simulink model "CryoDetXray"  (R2016b)
settings: Solver=ode45  StartTime=0.0  StopTime=10e-5  MaxStep=Tclk/4  RelTol=1e-3
values from neighbouring files (symbols this model uses):
  Fclk = Fadc    (= 307200000)    [setupCryoFPGAxray.m]
  Tclk = 1/Fclk    (= 3.25520833333e-09)    [setupCryoFPGAxray.m]
undefined symbols (not defined in the file or in its folder): AXI4, Lite, lpf, Naxi, xlipgetpartsetting
libraries: xbsIndex_r4 x1091, CryoDetLib x68, simulink x4, hdlsllib x1
(part 1 of 8)
settings Model: Creator=ssmith  LastModifiedBy=ssmith
settings DataIOCC: LimitDataPoints=on  SaveFormat=Array
settings OptimizationCC: BlockReduction=off  BooleanDataType=off  LifeSpan=inf
settings DebuggingCC: SaveWithParameterizedLinksMsg=none  UnderspecifiedInitializationDetection=Classic  MergeDetectMultiDrivingBlocksExec=none  SignalResolutionControl=TryResolveAllWithWarning  AllowSymbolicDim=off  SFUnexpectedBacktrackingDiag=warning  SFNoUnconditionalDefaultTransitionDiag=warning  SFExecutionAtInitializationDiag=none
settings HardwareCC: ProdBitPerPointer=32  ProdBitPerSizeT=32  ProdBitPerPtrDiffT=32  ProdLargestAtomicFloat=None  ProdIntDivRoundTo=Undefined  ProdEndianess=Unspecified  ProdWordSize=32  ProdHWDeviceType=32-bit Generic  TargetUnknown=on
settings ModelReferenceCC: PropagateSignalLabelsOutOfModel=off
settings GRTTargetCC: TargetLangStandard=C89/C90 (ANSI)  GeneratePreprocessorConditionals=Disable all
settings ConfigComp: CovMetricSettings=dw  CovHtmlReporting=on  CovSaveCumulativeToWorkspaceVar=on  CovSaveSingleToWorkspaceVar=on  CovExternalEMLEnable=off  CovSFcnEnable=off

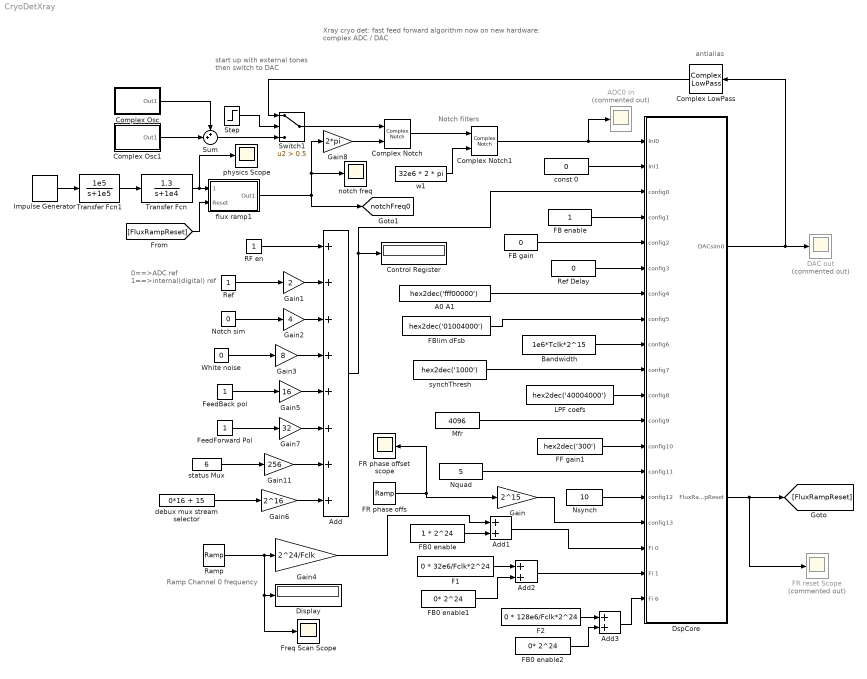
== system CryoDetXray ==
  note: antialias
  note: Ramp Channel 0 frequency
  note: Notch filters
  note: start up with external tones
      | then switch to DAC
  note: Xray cryo det: fast feed forward algorithm
      | now on new hardware:
      | complex ADC / DAC
  note: 0==>ADC ref
      | 1==>internal(digital) ref
  A0 A1 : Constant  Value=hex2dec('fff00000')  SampleTime=Tclk
  ADC0 in : Scope  Commented=on
  Add : Sum  Inputs=++++++++
  Add1 : Sum
  Add2 : Sum
  Add3 : Sum
  Bandwidth : Constant  Value=1e6*Tclk*2^15  SampleTime=Tclk
  Complex LowPass : CryoDetLib/Complex LowPass  num=lpf.num{1}  den=lpf.den{1}
  Complex Notch : CryoDetLib/Complex Notch  Q=16  depth=.95  Q1=10  depth1=1  Q2=10  depth2=1
  Complex Notch1 : CryoDetLib/Complex Notch  Q=8  depth=0.95  Q1=10  depth1=1  Q2=10  depth2=1
  Complex Osc : Subsystem  mask{Freq=64e6, Ampl=0.2}
  Complex Osc1 : Subsystem  mask{Freq=32e6, Ampl=0.2}
  Control Register : Display
      settings: Format=hex (Stored Integer)  Decimation=1000
  DAC out : Scope  Commented=on
  Display : Display
      settings: Decimation=64
  DspCore : Subsystem
  F1 : Constant  Value=0 * 32e6/Fclk*2^24  SampleTime=Tclk
  F2 : Constant  Value=0 * 128e6/Fclk*2^24  SampleTime=Tclk
  FB enable : Constant  SampleTime=Tclk
  FB gain : Constant  Value=0  SampleTime=Tclk
  FB0 enable : Constant  Value=1 * 2^24  SampleTime=Tclk
  FB0 enable1 : Constant  Value=0* 2^24  SampleTime=Tclk
  FB0 enable2 : Constant  Value=0* 2^24  SampleTime=Tclk
  FBlim dFsb : Constant  Value=hex2dec('01004000')  SampleTime=Tclk
  FF gain1 : Constant  Value=hex2dec('300')  SampleTime=Tclk
  FR phase offset scope : Scope
  FR phase offs : simulink/Sources/Ramp  slope=0/40e-5  start=26e-6  X0=.874
  FR reset Scope : Scope  Commented=on
  FeedBack pol : Constant  SampleTime=Tclk
  FeedForward Pol : Constant  SampleTime=Tclk
  Freq Scan Scope : Scope
  Gain : Gain  Gain=2^15
  Gain1 : Gain  Gain=2
  Gain11 : Gain  Gain=256
  Gain2 : Gain  Gain=4
  Gain3 : Gain  Gain=8
  Gain4 : Gain  Gain=2^24/Fclk
  Gain5 : Gain  Gain=16
  Gain6 : Gain  Gain=2^16
  Gain7 : Gain  Gain=32
  Gain8 : Gain  Gain=2*pi
  Impulse Generator : CryoDetLib/Impulse Generator  Impulse=1  width=2e-6  Period=1e-3  delay=15e-6
  LPF coefs : Constant  Value=hex2dec('40004000')  SampleTime=Tclk
  Mfr : Constant  Value=4096  SampleTime=Tclk
  Notch sim : Constant  Value=0  SampleTime=Tclk
  Nquad : Constant  Value=5  SampleTime=Tclk
  Nsynch : Constant  Value=10  SampleTime=Tclk
  RF en : Constant  SampleTime=Tclk
  Ramp : simulink/Sources/Ramp  slope=0 * 2e6/4e-6  start=1e-6  X0=64.0e6
  Ref : Constant  SampleTime=Tclk
  Ref Delay : Constant  Value=0  SampleTime=Tclk
  Step : Step  Time=2e-7  SampleTime=0
  Sum : Sum  Inputs=++|
  Switch1 : Switch  Criteria=u2 > Threshold  Threshold=0.5
  Transfer Fcn : TransferFcn  Numerator=[1.3]  Denominator=[1 1e4]
  Transfer Fcn1 : TransferFcn  Numerator=[1e5]  Denominator=[1 1e5]
  White noise : Constant  Value=0  SampleTime=Tclk
  const 0 : Constant  Value=0  SampleTime=Tclk
  debux mux stream selector : Constant  Value=0*16 + 15  SampleTime=Tclk
  flux ramp1 : Subsystem
  notch freq : Scope
  physics Scope : Scope
  status Mux : Constant  Value=6  SampleTime=Tclk
  synchThresh : Constant  Value=hex2dec('1000')  SampleTime=Tclk
  w1 : Constant  Value=32e6 * 2 * pi  SampleTime=Tclk
  tag scope: notchFreq0=global
  wires:
  Add/1 -> DspCore/3(config0), Control Register/1
  FB enable/1 -> DspCore/4(config1)
  DspCore/1(DACsim0) -> Complex LowPass/1, DAC out/1
  Sum/1 -> Switch1/3
  Step/1 -> Switch1/2
  RF en/1 -> Add/1
  Ref/1 -> Gain1/1
  Notch sim/1 -> Gain2/1
  White noise/1 -> Gain3/1
  FeedBack pol/1 -> Gain5/1
  debux mux stream selector/1 -> Gain6/1
  Gain1/1 -> Add/2
  Gain2/1 -> Add/3
  Gain3/1 -> Add/4
  status Mux/1 -> Gain11/1
  Complex Notch1/1 -> ADC0 in/1, DspCore/1(InI0)
  const 0/1 -> DspCore/2(InI1)
  Gain11/1 -> Add/7
  Gain6/1 -> Add/8
  Gain5/1 -> Add/5
  FB gain/1 -> DspCore/5(config2)
  Ref Delay/1 -> DspCore/6(config3)
  A0 A1/1 -> DspCore/7("config4 ")
  FBlim dFsb/1 -> DspCore/8(config5)
  Bandwidth/1 -> DspCore/9(config6)
  FeedForward Pol/1 -> Gain7/1
  FB0 enable/1 -> Add1/2
  Gain4/1 -> Add1/1
  Add1/1 -> DspCore/17(Fi 0)
  DspCore/2(FluxRampReset) -> [FluxRampReset], FR reset Scope/1
  Switch1/1 -> Complex Notch/1
  FB0 enable1/1 -> Add2/2
  F1/1 -> Add2/1
  Add2/1 -> DspCore/18(Fi 1)
  synchThresh/1 -> DspCore/10(config7)
  LPF coefs/1 -> DspCore/11(config8)
  FB0 enable2/1 -> Add3/2
  F2/1 -> Add3/1
  Add3/1 -> DspCore/19(Fi 6)
  Mfr/1 -> DspCore/12(config9)
  FF gain1/1 -> DspCore/13(config10)
  Nquad/1 -> DspCore/14(config11)
  Nsynch/1 -> DspCore/15(config12)
  Complex Osc1/1(Out1) -> Sum/2
  Complex Osc/1(Out1) -> Sum/1
  Gain8/1 -> Complex Notch/2
  w1/1 -> Complex Notch1/2
  [FluxRampReset] -> flux ramp1/2(Reset)
  Gain/1 -> DspCore/16(config13)
  Gain7/1 -> Add/6
  Ramp/1 -> Freq Scan Scope/1, Display/1, Gain4/1
  Impulse Generator/1 -> Transfer Fcn1/1
  Transfer Fcn/1 -> physics Scope/1, flux ramp1/1(physics)
  Complex LowPass/1 -> Switch1/1
  Complex Notch/1 -> Complex Notch1/1
  FR phase offs/1 -> Gain/1, FR phase offset scope/1
  flux ramp1/1(Out1) -> [notchFreq0], Gain8/1, notch freq/1
  Transfer Fcn1/1 -> Transfer Fcn/1

== system CryoDetXray/Complex Osc ==
  Cosine : Sin  Amplitude=Ampl  Frequency=2*pi*Freq  Phase=pi/2  SampleTime=0
  Real-Imag to Complex : RealImagToComplex
  Sine : Sin  Amplitude=Ampl  Frequency=2*pi*Freq  SampleTime=0
  Out1 : Outport
  wires:
  Real-Imag to Complex/1 -> Out1/1
  Cosine/1 -> Real-Imag to Complex/1
  Sine/1 -> Real-Imag to Complex/2

== system CryoDetXray/Complex Osc1 ==
  Cosine : Sin  Amplitude=Ampl  Frequency=2*pi*Freq  Phase=pi/2  SampleTime=0
  Real-Imag to Complex : RealImagToComplex
  Sine : Sin  Amplitude=Ampl  Frequency=2*pi*Freq  SampleTime=0
  Out1 : Outport
  wires:
  Real-Imag to Complex/1 -> Out1/1
  Cosine/1 -> Real-Imag to Complex/1
  Sine/1 -> Real-Imag to Complex/2

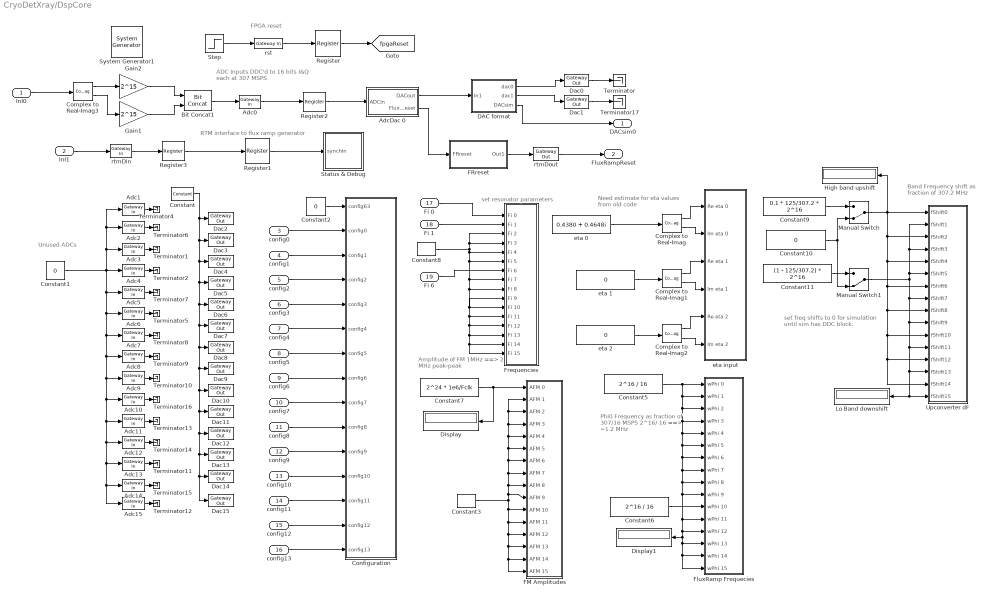
== system CryoDetXray/DspCore ==
  note: set freq shifts to 0 for simulation
      | until sim has DDC block.
  note: RTM interface to flux ramp generator
  note: Need estimate for eta values
      | from old code
  note: set resonator parameters
  note: Phi0 Frequency as fraction of 307/16 MSPS
      | 2^16/ 16 ==> ~1.2 MHz
  note: Amplitude of FM
      | 1MHz ==>
      | 2 MHz peak-peak
  note: Unused ADCs
  note: ADC Inputs DDC'd to
      | 16 bits I&Q each at 307 MSPS
  note: FPGA reset
  note: Band Frequency shift as fraction of 307.2 MHz
  InI0 : Inport
  InI1 : Inport  Port=2
  config0 : Inport  Port=3
  config1 : Inport  Port=4
  config2 : Inport  Port=5
  config3 : Inport  Port=6
  "config4 " : Inport  Port=7
  config5 : Inport  Port=8
  config6 : Inport  Port=9
  config7 : Inport  Port=10
  config8 : Inport  Port=11
  config9 : Inport  Port=12
  config10 : Inport  Port=13
  config11 : Inport  Port=14
  config12 : Inport  Port=15
  config13 : Inport  Port=16
  Fi 0 : Inport  Port=17
  Fi 1 : Inport  Port=18
  Fi 6 : Inport  Port=19
  " System Generator1" : xbsIndex_r4/ System Generator  Tag=genX  xilinxfamily=kintexu  part=xcku060  speed=-2-e  package=ffva1156  synthesis_tool=Vivado  clock_wrapper=Clock Enables  directory=./netlist  proj_type=Vivado  Synth_file=Vivado Synthesis Defaults  Impl_file=Vivado Implementation Defaults  testbench=off  simulink_period=Tclk  sysclk_period=Tclk*1e9  dcm_input_clock_period=10  incr_netlist=off  trim_vbits=Everywhere in SubSystem  dbl_ovrd=According to Block Masks  core_generation=According to Block Masks  run_coregen=off  deprecated_control=off  eval_field=0  block_type=sysgen
  Adc{0..15} (16 alike) : xbsIndex_r4/Gateway In  gui_display_data_type=Fixed-point  arith_type=Unsigned  n_bits=32  bin_pt=0  preci_type=Single  exp_width=8  frac_width=24  rows=1  columns=1  quantization=Truncate  overflow=Wrap  period=Ts  UseAsADC=off  ADCChannel='1'  interface=None  automatic_assignment=on  address_offset=hex2dec('00')  intf_name=''  intf_description=''  default_value=0  timing_constraint=None  locs_specified=off  LOCs={}  io_standard={}  inherit_from_input=off  hdl_port=on  dbl_ovrd=off  block_type=gatewayin
  AdcDac 0 : Subsystem
  Bit Concat1 : hdlsllib/HDL Operations/Bit Concat  numInputs=2
  Complex to Real-Imag{,1..3} (4 alike) : ComplexToRealImag
  Configuration : Subsystem
  Constant : xbsIndex_r4/Constant  const=0  gui_display_data_type=Fixed-point  arith_type=Unsigned  n_bits=32  bin_pt=0  preci_type=Single  exp_width=8  frac_width=24  explicit_period=off  period=1  equ=P=C  opselect=C  inp2=PCIN>>17  opr=+  inp1=P  carry=CIN  dbl_ovrd=off  block_type=constant
  Constant1 : Constant  Value=0
  Constant10 : Constant  Value=0
  Constant11 : Constant  Value=(1 - 125/307.2) * 2^16
  Constant2 : Constant  Value=0
  Constant3 : xbsIndex_r4/Constant  const=0  gui_display_data_type=Fixed-point  arith_type=Unsigned  n_bits=32  bin_pt=0  preci_type=Single  exp_width=8  frac_width=24  explicit_period=on  period=Tclk*Naxi  equ=P=C  opselect=C  inp2=PCIN>>17  opr=+  inp1=P  carry=CIN  dbl_ovrd=off  block_type=constant
  Constant5 : Constant  Value=2^16 / 16
  Constant6 : Constant  Value=2^16 / 16
  Constant7 : Constant  Value=2^24 * 1e6/Fclk
  Constant8 : xbsIndex_r4/Constant  const=0  gui_display_data_type=Fixed-point  arith_type=Unsigned  n_bits=32  bin_pt=0  preci_type=Single  exp_width=8  frac_width=24  explicit_period=on  period=Tclk*Naxi  equ=P=C  opselect=C  inp2=PCIN>>17  opr=+  inp1=P  carry=CIN  dbl_ovrd=off  block_type=constant
  Constant9 : Constant  Value="0.1  * 125/307.2 * 2^16"
  DAC format : Subsystem
  Dac{0,2..15} (15 alike) : xbsIndex_r4/Gateway Out  inherit_from_input=on  hdl_port=on  rows=1  columns=1  UseAsDAC=off  DACChannel='1'  interface=None  automatic_assignment=on  address_offset=hex2dec('00')  intf_name=''  intf_description=''  timing_constraint=None  locs_specified=off  LOCs={}  io_standard={}  block_type=gatewayout
  "Dac1 " : xbsIndex_r4/Gateway Out  inherit_from_input=on  hdl_port=on  rows=1  columns=1  UseAsDAC=off  DACChannel='1'  interface=None  automatic_assignment=on  address_offset=hex2dec('00')  intf_name=''  intf_description=''  timing_constraint=None  locs_specified=off  LOCs={}  io_standard={}  block_type=gatewayout
  Display : Display
  Display1 : Display
  FM Amplitudes : Subsystem
  FRreset : Subsystem
  FluxRamp Frequecies : Subsystem
  Frequencies : Subsystem
  Gain1 : Gain  Gain=2^15  OutDataTypeStr=int16  RndMeth=Nearest  SaturateOnIntegerOverflow=on
  Gain2 : Gain  Gain=2^15  OutDataTypeStr=int16  RndMeth=Nearest  SaturateOnIntegerOverflow=on
  High band upshift : Display
  Lo Band downshift : Display
  Manual Switch : ManualSwitch  CurrentSetting=0
  Manual Switch1 : ManualSwitch  CurrentSetting=0
  Register : xbsIndex_r4/Register  init=1  rst=off  en=off  dbl_ovrd=off  block_type=register
  Register1 : xbsIndex_r4/Register  init=1  rst=off  en=off  dbl_ovrd=off  block_type=register
  Register2 : xbsIndex_r4/Register  init=0  rst=off  en=off  dbl_ovrd=off  block_type=register
  Register3 : xbsIndex_r4/Register  init=0  rst=off  en=off  dbl_ovrd=off  block_type=register
  Status & Debug : Subsystem
  Step : Step  Time=1e-7  Before=1  After=0  SampleTime=0
  Terminator{,1..2,4..17} (17 alike) : Terminator
  Upconverter dF : Subsystem
  eta 0 : Constant  Value=0.4380 + 0.4648i
  eta 1 : Constant  Value=0
  "eta 2 " : Constant  Value=0
  eta input : Subsystem
  rst : xbsIndex_r4/Gateway In  gui_display_data_type=Boolean  arith_type=Boolean  n_bits=16  bin_pt=14  preci_type=Single  exp_width=8  frac_width=24  rows=1  columns=1  quantization="Round  (unbiased: +/- Inf)"  overflow=Saturate  period=Tclk  UseAsADC=off  ADCChannel='1'  interface=None  automatic_assignment=on  address_offset=hex2dec('00')  intf_name=''  intf_description=''  default_value=0  timing_constraint=None  locs_specified=off  LOCs={}  io_standard={}  inherit_from_input=off  hdl_port=on  dbl_ovrd=off  block_type=gatewayin
  rtmDin : xbsIndex_r4/Gateway In  gui_display_data_type=Fixed-point  arith_type=Unsigned  n_bits=16  bin_pt=0  preci_type=Single  exp_width=8  frac_width=24  rows=1  columns=1  quantization=Truncate  overflow=Wrap  period=Tclk  UseAsADC=off  ADCChannel='1'  interface=None  automatic_assignment=on  address_offset=hex2dec('00')  intf_name=''  intf_description=''  default_value=0  timing_constraint=None  locs_specified=off  LOCs={}  io_standard={}  inherit_from_input=off  hdl_port=on  dbl_ovrd=off  block_type=gatewayin
  rtmDout : xbsIndex_r4/Gateway Out  inherit_from_input=off  hdl_port=on  rows=1  columns=1  UseAsDAC=off  DACChannel='1'  interface=None  automatic_assignment=on  address_offset=hex2dec('00')  intf_name=''  intf_description=''  timing_constraint=None  locs_specified=off  LOCs={}  io_standard={}  block_type=gatewayout
  DACsim0 : Outport
  FluxRampReset : Outport  Port=2
  tag scope: fpgaReset=global
  wires:
  Step/1 -> rst/1
  rst/1 -> Register/1
  config0/1 -> Configuration/2(config0)
  config1/1 -> Configuration/3(config1)
  config2/1 -> Configuration/4(config2)
  config3/1 -> Configuration/5(config3)
  "config4 "/1 -> Configuration/6(config4)
  config5/1 -> Configuration/7(config5)
  config6/1 -> Configuration/8(config6)
  Fi 0/1 -> Frequencies/1("Fi 0 ")
  Register/1 -> [fpgaReset]
  Constant2/1 -> Configuration/1(config63)
  Fi 1/1 -> Frequencies/2(Fi 1)
  config7/1 -> Configuration/9(config7)
  config8/1 -> Configuration/10(config8)
  config9/1 -> Configuration/11(config9)
  config10/1 -> Configuration/12(config10)
  config11/1 -> Configuration/13(config11)
  config12/1 -> Configuration/14(config12)
  Constant8/1 -> Frequencies/3(Fi 2), Frequencies/4(Fi 3), Frequencies/16(Fi 15), Frequencies/15(Fi 14), Frequencies/14(Fi 13), Frequencies/13(Fi 12), Frequencies/12(Fi 11), Frequencies/11(Fi 10), Frequencies/10(Fi 9), Frequencies/9(Fi 8), Frequencies/8(Fi 7), Frequencies/6(Fi 5), Frequencies/5(Fi 4)
  Fi 6/1 -> Frequencies/7(Fi 6)
  AdcDac 0/2(FluxRampReset) -> FRreset/1(FRreset)
  Complex to Real-Imag/1 -> eta input/1(Re eta 0)
  Complex to Real-Imag/2 -> eta input/2(Im eta 0)
  Complex to Real-Imag1/1 -> eta input/3(Re eta 1)
  Complex to Real-Imag1/2 -> eta input/4(Im eta 1)
  eta 1/1 -> Complex to Real-Imag1/1
  Complex to Real-Imag2/1 -> eta input/5(Re eta 2)
  Complex to Real-Imag2/2 -> eta input/6(Im eta 2)
  "eta 2 "/1 -> Complex to Real-Imag2/1
  Constant6/1 -> FluxRamp Frequecies/11(wPhi 10)
  Constant7/1 -> Display/1, FM Amplitudes/1(AFM 0)
  Adc0/1 -> Register2/1
  FRreset/1(Out1) -> rtmDout/1
  Dac0/1 -> Terminator/1
  rtmDout/1 -> FluxRampReset/1
  Gain2/1 -> Bit Concat1/1
  Gain1/1 -> Bit Concat1/2
  Bit Concat1/1 -> Adc0/1
  config13/1 -> Configuration/15(config13)
  eta 0/1 -> Complex to Real-Imag/1
  Constant3/1 -> FM Amplitudes/11(AFM 10), FM Amplitudes/12(AFM 11), FM Amplitudes/13(AFM 12), FM Amplitudes/14(AFM 13), FM Amplitudes/15(AFM 14), FM Amplitudes/16(AFM 15), FM Amplitudes/10(AFM 9), FM Amplitudes/2(AFM 1), FM Amplitudes/3(AFM 2), FM Amplitudes/4(AFM 3), FM Amplitudes/5(AFM 4), FM Amplitudes/6(AFM 5), FM Amplitudes/7(AFM 6), FM Amplitudes/8(AFM 7), FM Amplitudes/9(AFM 8)
  Constant5/1 -> FluxRamp Frequecies/2(wPhi 1), FluxRamp Frequecies/3(wPhi 2), FluxRamp Frequecies/4(wPhi 3), FluxRamp Frequecies/5(wPhi 4), FluxRamp Frequecies/6(wPhi 5), FluxRamp Frequecies/7(wPhi 6), FluxRamp Frequecies/8(wPhi 7), FluxRamp Frequecies/13(wPhi 12), FluxRamp Frequecies/14(wPhi 13), FluxRamp Frequecies/15(wPhi 14), FluxRamp Frequecies/16(wPhi 15), Display1/1, FluxRamp Frequecies/12(wPhi 11), FluxRamp Frequecies/10(wPhi 9), FluxRamp Frequecies/9(wPhi 8), FluxRamp Frequecies/1(wPhi 0)
  Constant1/1 -> Adc5/1, Adc7/1, Adc8/1, Adc9/1, Adc10/1, Adc11/1, Adc12/1, Adc13/1, Adc14/1, Adc15/1, Adc6/1, Adc4/1, Adc3/1, Adc1/1, Adc2/1
  Complex to Real-Imag3/1 -> Gain2/1
  InI0/1 -> Complex to Real-Imag3/1
  Complex to Real-Imag3/2 -> Gain1/1
  InI1/1 -> rtmDin/1
  Adc6/1 -> Terminator5/1
  Adc7/1 -> Terminator8/1
  Adc8/1 -> Terminator9/1
  Adc9/1 -> Terminator10/1
  Adc11/1 -> Terminator13/1
  Adc12/1 -> Terminator14/1
  Adc13/1 -> Terminator11/1
  Adc14/1 -> Terminator15/1
  Adc15/1 -> Terminator12/1
  Adc10/1 -> Terminator16/1
  Adc1/1 -> Terminator4/1
  Adc2/1 -> Terminator6/1
  Adc3/1 -> Terminator1/1
  Adc4/1 -> Terminator2/1
  Adc5/1 -> Terminator7/1
  AdcDac 0/1(DACout) -> DAC format/1(In1)
  DAC format/3(DACsim) -> DACsim0/1
  DAC format/1(dac0) -> Dac0/1
  DAC format/2(dac1) -> "Dac1 "/1
  "Dac1 "/1 -> Terminator17/1
  Constant/1 -> Dac4/1, Dac5/1, Dac6/1, Dac7/1, Dac8/1, Dac9/1, Dac10/1, Dac11/1, Dac12/1, Dac13/1, Dac14/1, Dac15/1, Dac3/1, Dac2/1
  Manual Switch/1 -> Upconverter dF/1(fShift0), Upconverter dF/3(fShift2), Upconverter dF/5(fShift4), Upconverter dF/7(fShift6), Upconverter dF/11(fShift10), Upconverter dF/13(fShift12), Upconverter dF/15(fShift14), Upconverter dF/9(fShift8), High band upshift/1
  Constant9/1 -> Manual Switch/1
  Constant10/1 -> Manual Switch/2, Manual Switch1/2
  Constant11/1 -> Manual Switch1/1
  Manual Switch1/1 -> Upconverter dF/8(fShift7), Upconverter dF/10(fShift9), Upconverter dF/12(fShift11), Upconverter dF/14(fShift13), Lo Band downshift/1, Upconverter dF/16(fShift15), Upconverter dF/4(fShift3), Upconverter dF/2(fShift1), Upconverter dF/6(fShift5)
  rtmDin/1 -> Register3/1
  Register1/1 -> Status & Debug/1(synchIn)
  Register3/1 -> Register1/1
  Register2/1 -> AdcDac 0/1(ADCin)

== system CryoDetXray/flux ramp1 ==
  note: Simulate flux-ramp modulated center frequency of notch
      | with reset from flux ramp reset
  physics : Inport
  Reset : Inport  Port=2
  Add : Sum  Inputs=++|
  Add4 : Sum
  F1 : Constant  Value=307.2e6 / 16 / 16
  F3 : Constant  Value=64e6
  Integrator : Integrator  ExternalReset=rising
  Resonator w Flux Ramp Scope : Scope  Commented=on
  Resonator w Flux Ramp Scope1 : Scope  Commented=on
  Sine Wave : Sin  TimeSource=Use external signal  Amplitude=1e6  Frequency=2*pi  SampleTime=0
  Out1 : Outport
  wires:
  Add4/1 -> Resonator w Flux Ramp Scope/1, Out1/1
  F3/1 -> Add4/2
  F1/1 -> Integrator/1
  Reset/1 -> Integrator/2
  Sine Wave/1 -> Add4/1
  Integrator/1 -> Add/2
  Add/1 -> Resonator w Flux Ramp Scope1/1, Sine Wave/1
  physics/1 -> Add/1

== system CryoDetXray/DspCore/AdcDac 0 ==
  note: commented out 7 Oct 2017 as LR says number of logic level too much for router
  note: Does NOT work yet
      | 26 Sep 2017
  note: loop filter for loop which feeds back on
      | phase of flux ramp
  note: Estimate FluxRamp Phase
  note: Estimate frequency error at high bandwidth
  note: freqBusHBW goes to DDS to generate output tones
      | FR reset goes to flux ramp function generator
  note: loop filter output will be mux'd channel, fluix ramp phase shift
  note: High bandwidth/ no sideband scheme
  note: Low Bandwidth / +- sideband scheme
      | (but sideband generator has been removed)
  note: 9 June SRS pulled LPF out of eta subsytem
      | so that amplitudes subsystem can use low-pass filtered I&Q data
      | Also added Signal central line to LPF processing as Amplitudes block uses it, though eta does not
  ADCin : Inport
  16LineUDC 0 : Subsystem
  16LineUDC 1 : Subsystem
  16ch LBW LPF : Subsystem
  Amplitudes : Subsystem
  Bus Creator : BusCreator  Inputs=2
  Bus Selector : BusSelector  Commented=on  OutputSignals=channel,Sig&Ref.SignalQ&I.sigQ,Sig&Ref.SignalQ&I.sigI,Sig&Ref.ReferenceQ&I.refQ,Sig&Ref.ReferenceQ&I.refI
  "Flux Ramp DDC " : Subsystem
  FluxRamp : Subsystem
  Gateway Out{1..3,5..6} (5 alike) : xbsIndex_r4/Gateway Out  Commented=on  inherit_from_input=off  hdl_port=off  rows=1  columns=1  UseAsDAC=off  DACChannel='1'  interface=None  automatic_assignment=on  address_offset=hex2dec('00')  intf_name=''  intf_description=''  timing_constraint=None  locs_specified=off  LOCs={}  io_standard={}  block_type=gatewayout
  HBW Sig/Ref LPF : Subsystem  Commented=on
  Mux : Mux  Commented=on  Inputs=2
  Mux1 : Mux  Commented=on  Inputs=2
  RF switch : Subsystem
  Ref Delay : Subsystem
  S21 : Subsystem  Commented=on
  SigXrefIQ : Scope  Commented=on  NumInputPorts=3
  Terminator : Terminator
  Terminator2 : Terminator  Commented=on
  Terminator3 : Terminator  Commented=on
  dF1 : Subsystem
  dphi : Subsystem
  loopFilter1 : Subsystem
  shiftFreq : Subsystem
  DACout : Outport
  FluxRampReset : Outport  Port=2
  tag scope: freqBusHBW=global
  wires:
  16LineUDC 1/1(Out1) -> Terminator/1
  16LineUDC 0/1(toDAC) -> RF switch/1(In1)
  ADCin/1 -> Bus Creator/1  "ADCin"
  Ref Delay/1(Out1) -> Bus Creator/2
  Bus Creator/1 -> 16LineUDC 1/1(In1), 16LineUDC 0/1(In1)
  16LineUDC 0/2(demodulated) -> 16ch LBW LPF/1(In1)
  RF switch/1(Out1) -> Ref Delay/1(In1), shiftFreq/1(In1)
  16ch LBW LPF/1(Out1) -> Amplitudes/1(In2)
  16LineUDC 0/3(hiBW) -> Bus Selector/1, HBW Sig/Ref LPF/1(In1), dF1/1(In1)
  HBW Sig/Ref LPF/1(Out1) -> S21/1(In2)
  loopFilter1/1(Out1) -> FluxRamp/1(phiFR)
  "Flux Ramp DDC "/1(Out1) -> loopFilter1/1(In1)
  FluxRamp/2(freqBusHBW) -> [freqBusHBW]
  FluxRamp/4(FiBus) -> dphi/1(In1)
  FluxRamp/3(FR reset) -> FluxRampReset/1
  S21/1(S21Bus) -> Terminator2/1
  S21/2(S21BusLPF) -> Terminator3/1
  dF1/1(Out1) -> "Flux Ramp DDC "/1(FreqErrIn)
  FluxRamp/1(FluxRampLO) -> "Flux Ramp DDC "/2(FluxRampLO)
  shiftFreq/1(Out1) -> DACout/1
  Gateway Out5/1 -> Mux/1
  Gateway Out6/1 -> Mux/2
  Gateway Out2/1 -> Mux1/2
  Gateway Out1/1 -> Mux1/1
  Gateway Out3/1 -> SigXrefIQ/1
  Mux/1 -> SigXrefIQ/2
  Mux1/1 -> SigXrefIQ/3
  Bus Selector/1 -> Gateway Out3/1  "<channel>"
  Bus Selector/2 -> Gateway Out5/1  "<sigQ>"
  Bus Selector/3 -> Gateway Out6/1  "<sigI>"
  Bus Selector/4 -> Gateway Out1/1  "<refQ>"
  Bus Selector/5 -> Gateway Out2/1  "<refI>"

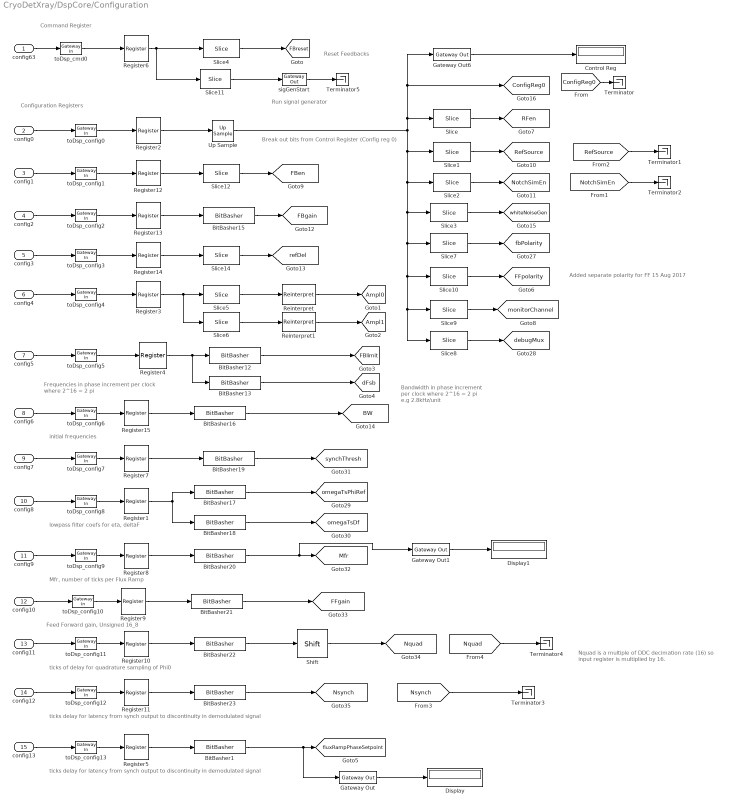
== system CryoDetXray/DspCore/Configuration ==
  note: Run signal generator
  note: Reset Feedbacks
  note: Nquad is a multiple of DDC decimation rate (16)
      | so input register is multiplied by 16.
  note: Added separate polarity for FF 15 Aug 2017
  note: Frequencies in phase increment per clock
      | where 2^16 = 2 pi
  note: initial frequencies
  note: Configuration Registers
  note: Command Register
  note: Break out bits from Control Register (Config reg 0)
  note: Bandwidth in phase increment per clock
      | where 2^16 = 2 pi e.g 2.8kHz/unit
  note: lowpass filter coefs for eta, deltaF
  note: Mfr, number of ticks per Flux Ramp
  note: Feed Forward gain, Unsigned 16_8
  note: ticks of delay for quadrature sampling of Phi0
  note: ticks delay for latency from synch output to discontinuity in demodulated signal
  note: ticks delay for latency from synch output to discontinuity in demodulated signal
  config63 : Inport
  config0 : Inport  Port=2
  config1 : Inport  Port=3
  config2 : Inport  Port=4
  config3 : Inport  Port=5
  config4 : Inport  Port=6
  config5 : Inport  Port=7
  config6 : Inport  Port=8
  config7 : Inport  Port=9
  config8 : Inport  Port=10
  config9 : Inport  Port=11
  config10 : Inport  Port=12
  config11 : Inport  Port=13
  config12 : Inport  Port=14
  config13 : Inport  Port=15
  BitBasher1 : xbsIndex_r4/BitBasher  bitexpr=a={b[15:0]}  display_expr=on  sr_1=a  arith_type1="Signed  (2's comp)"  bin_pt1=15  sr_2=2  arith_type2=Unsigned  bin_pt2=0  sr_3=3  arith_type3=Unsigned  bin_pt3=0  sr_4=4  arith_type4=Unsigned  bin_pt4=0  dbl_ovrd=off  block_type=bitbasher
  BitBasher12 : xbsIndex_r4/BitBasher  bitexpr=a={b[31:16]}  display_expr=on  sr_1=a  arith_type1=Unsigned  bin_pt1=16  sr_2=2  arith_type2=Unsigned  bin_pt2=0  sr_3=3  arith_type3=Unsigned  bin_pt3=0  sr_4=4  arith_type4=Unsigned  bin_pt4=0  dbl_ovrd=off  block_type=bitbasher
  BitBasher13 : xbsIndex_r4/BitBasher  bitexpr=a={b[15:0]}  display_expr=on  sr_1=a  arith_type1=Unsigned  bin_pt1=16  sr_2=2  arith_type2=Unsigned  bin_pt2=0  sr_3=3  arith_type3=Unsigned  bin_pt3=0  sr_4=4  arith_type4=Unsigned  bin_pt4=0  dbl_ovrd=off  block_type=bitbasher
  BitBasher15 : xbsIndex_r4/BitBasher  bitexpr=a={b[15:0]}  display_expr=on  sr_1=a  arith_type1=Unsigned  bin_pt1=12  sr_2=2  arith_type2=Unsigned  bin_pt2=0  sr_3=3  arith_type3=Unsigned  bin_pt3=0  sr_4=4  arith_type4=Unsigned  bin_pt4=0  dbl_ovrd=off  block_type=bitbasher
  BitBasher16 : xbsIndex_r4/BitBasher  bitexpr=a={b[15:0]}  display_expr=on  sr_1=a  arith_type1="Signed  (2's comp)"  bin_pt1=15  sr_2=2  arith_type2=Unsigned  bin_pt2=0  sr_3=3  arith_type3=Unsigned  bin_pt3=0  sr_4=4  arith_type4=Unsigned  bin_pt4=0  dbl_ovrd=off  block_type=bitbasher
  BitBasher17 : xbsIndex_r4/BitBasher  bitexpr=a={b[15:0]}  display_expr=on  sr_1=a  arith_type1=Unsigned  bin_pt1=16  sr_2=2  arith_type2=Unsigned  bin_pt2=0  sr_3=3  arith_type3=Unsigned  bin_pt3=0  sr_4=4  arith_type4=Unsigned  bin_pt4=0  dbl_ovrd=off  block_type=bitbasher
  BitBasher18 : xbsIndex_r4/BitBasher  bitexpr=a={b[31:16]}  display_expr=on  sr_1=a  arith_type1=Unsigned  bin_pt1=16  sr_2=2  arith_type2=Unsigned  bin_pt2=0  sr_3=3  arith_type3=Unsigned  bin_pt3=0  sr_4=4  arith_type4=Unsigned  bin_pt4=0  dbl_ovrd=off  block_type=bitbasher
  BitBasher19 : xbsIndex_r4/BitBasher  bitexpr=a={b[15:0]}  display_expr=on  sr_1=a  arith_type1="Signed  (2's comp)"  bin_pt1=15  sr_2=2  arith_type2=Unsigned  bin_pt2=0  sr_3=3  arith_type3=Unsigned  bin_pt3=0  sr_4=4  arith_type4=Unsigned  bin_pt4=0  dbl_ovrd=off  block_type=bitbasher
  BitBasher20 : xbsIndex_r4/BitBasher  bitexpr=a={b[15:0]}  display_expr=on  sr_1=a  arith_type1=Unsigned  bin_pt1=0  sr_2=2  arith_type2=Unsigned  bin_pt2=0  sr_3=3  arith_type3=Unsigned  bin_pt3=0  sr_4=4  arith_type4=Unsigned  bin_pt4=0  dbl_ovrd=off  block_type=bitbasher
  BitBasher21 : xbsIndex_r4/BitBasher  bitexpr=a={b[15:0]}  display_expr=on  sr_1=a  arith_type1=Unsigned  bin_pt1=4  sr_2=2  arith_type2=Unsigned  bin_pt2=0  sr_3=3  arith_type3=Unsigned  bin_pt3=0  sr_4=4  arith_type4=Unsigned  bin_pt4=0  dbl_ovrd=off  block_type=bitbasher
  BitBasher22 : xbsIndex_r4/BitBasher  bitexpr=a={b[3:0]}  display_expr=on  sr_1=a  arith_type1=Unsigned  bin_pt1=0  sr_2=2  arith_type2=Unsigned  bin_pt2=0  sr_3=3  arith_type3=Unsigned  bin_pt3=0  sr_4=4  arith_type4=Unsigned  bin_pt4=0  dbl_ovrd=off  block_type=bitbasher
  BitBasher23 : xbsIndex_r4/BitBasher  bitexpr=a={b[7:0]}  display_expr=on  sr_1=a  arith_type1=Unsigned  bin_pt1=0  sr_2=2  arith_type2=Unsigned  bin_pt2=0  sr_3=3  arith_type3=Unsigned  bin_pt3=0  sr_4=4  arith_type4=Unsigned  bin_pt4=0  dbl_ovrd=off  block_type=bitbasher
  Control Reg : Display
  Display : Display
  Display1 : Display
  Gateway Out : xbsIndex_r4/Gateway Out  inherit_from_input=off  hdl_port=off  rows=1  columns=1  UseAsDAC=off  DACChannel='1'  interface=None  automatic_assignment=on  address_offset=hex2dec('00')  intf_name=''  intf_description=''  timing_constraint=None  locs_specified=off  LOCs={}  io_standard={}  block_type=gatewayout
  Gateway Out1 : xbsIndex_r4/Gateway Out  inherit_from_input=off  hdl_port=off  rows=1  columns=1  UseAsDAC=off  DACChannel='1'  interface=None  automatic_assignment=on  address_offset=hex2dec('00')  intf_name=''  intf_description=''  timing_constraint=None  locs_specified=off  LOCs={}  io_standard={}  block_type=gatewayout
  Gateway Out6 : xbsIndex_r4/Gateway Out  inherit_from_input=off  hdl_port=off  rows=1  columns=1  UseAsDAC=off  DACChannel='1'  interface=None  automatic_assignment=on  address_offset=hex2dec('00')  intf_name=''  intf_description=''  timing_constraint=None  locs_specified=off  LOCs={}  io_standard={}  block_type=gatewayout
  Register{1..15} (15 alike) : xbsIndex_r4/Register  init=0  rst=off  en=off  dbl_ovrd=off  block_type=register
  Reinterpret : xbsIndex_r4/Reinterpret  force_arith_type=on  arith_type=Unsigned  force_bin_pt=on  bin_pt=16  block_type=reinterpret
  Reinterpret1 : xbsIndex_r4/Reinterpret  force_arith_type=on  arith_type=Unsigned  force_bin_pt=on  bin_pt=16  block_type=reinterpret
  Shift : xbsIndex_r4/Shift  shift_dir=Left  shift_bits=4  en=off  latency=1  precision=User Defined  arith_type=Unsigned  n_bits=8  bin_pt=0  quantization=Truncate  overflow=Wrap  dbl_ovrd=off  block_type=shift
  Slice : xbsIndex_r4/Slice  nbits=1  boolean_output=off  mode=Upper Bit Location + Width  bit1=0  base1=LSB of Input  bit0=0  base0=LSB of Input  dbl_ovrd=off  block_type=slice
  Slice1 : xbsIndex_r4/Slice  nbits=1  boolean_output=on  mode=Upper Bit Location + Width  bit1=1  base1=LSB of Input  bit0=0  base0=LSB of Input  dbl_ovrd=off  block_type=slice
  Slice10 : xbsIndex_r4/Slice  nbits=1  boolean_output=on  mode=Upper Bit Location + Width  bit1=5  base1=LSB of Input  bit0=0  base0=LSB of Input  dbl_ovrd=off  block_type=slice
  Slice11 : xbsIndex_r4/Slice  nbits=1  boolean_output=on  mode=Upper Bit Location + Width  bit1=4  base1=LSB of Input  bit0=0  base0=LSB of Input  dbl_ovrd=off  block_type=slice
  Slice12 : xbsIndex_r4/Slice  nbits=1  boolean_output=on  mode=Upper Bit Location + Width  bit1=0  base1=LSB of Input  bit0=0  base0=LSB of Input  dbl_ovrd=off  block_type=slice
  Slice14 : xbsIndex_r4/Slice  nbits=8  boolean_output=off  mode=Lower Bit Location + Width  bit1=0  base1=LSB of Input  bit0=0  base0=LSB of Input  dbl_ovrd=off  block_type=slice
  Slice2 : xbsIndex_r4/Slice  nbits=1  boolean_output=on  mode=Upper Bit Location + Width  bit1=2  base1=LSB of Input  bit0=0  base0=LSB of Input  dbl_ovrd=off  block_type=slice
  Slice3 : xbsIndex_r4/Slice  nbits=1  boolean_output=on  mode=Upper Bit Location + Width  bit1=3  base1=LSB of Input  bit0=0  base0=LSB of Input  dbl_ovrd=off  block_type=slice
  Slice4 : xbsIndex_r4/Slice  nbits=1  boolean_output=on  mode=Upper Bit Location + Width  bit1=0  base1=LSB of Input  bit0=0  base0=LSB of Input  dbl_ovrd=off  block_type=slice
  Slice5 : xbsIndex_r4/Slice  nbits=16  boolean_output=off  mode=Upper Bit Location + Width  bit1=31  base1=LSB of Input  bit0=0  base0=LSB of Input  dbl_ovrd=off  block_type=slice
  Slice6 : xbsIndex_r4/Slice  nbits=16  boolean_output=off  mode=Upper Bit Location + Width  bit1=15  base1=LSB of Input  bit0=0  base0=LSB of Input  dbl_ovrd=off  block_type=slice
  Slice7 : xbsIndex_r4/Slice  nbits=1  boolean_output=on  mode=Upper Bit Location + Width  bit1=4  base1=LSB of Input  bit0=0  base0=LSB of Input  dbl_ovrd=off  block_type=slice
  Slice8 : xbsIndex_r4/Slice  nbits=8  boolean_output=off  mode=Lower Bit Location + Width  bit1=6  base1=LSB of Input  bit0=16  base0=LSB of Input  dbl_ovrd=off  block_type=slice
  Slice9 : xbsIndex_r4/Slice  nbits=8  boolean_output=off  mode=Lower Bit Location + Width  bit1=6  base1=LSB of Input  bit0=8  base0=LSB of Input  dbl_ovrd=off  block_type=slice
  Terminator{,1..5} (6 alike) : Terminator
  Up Sample : xbsIndex_r4/Up Sample  sample_ratio=Naxi  copy_samples=on  en=off  latency=1  dbl_ovrd=off  block_type=usamp
  sigGenStart : xbsIndex_r4/Gateway Out  inherit_from_input=on  hdl_port=on  rows=1  columns=1  UseAsDAC=off  DACChannel='1'  interface=None  automatic_assignment=off  address_offset=hex2dec('004')  intf_name=''  intf_description=''  timing_constraint=None  locs_specified=off  LOCs={}  io_standard={}  block_type=gatewayout
  toDsp_cmd0 : xbsIndex_r4/Gateway In  gui_display_data_type=Fixed-point  arith_type=Unsigned  n_bits=32  bin_pt=0  preci_type=Single  exp_width=8  frac_width=24  rows=1  columns=1  quantization=Truncate  overflow=Wrap  period=Tclk*Naxi  UseAsADC=off  ADCChannel='1'  interface=AXI4-Lite  automatic_assignment=off  address_offset=hex2dec('8fc')  intf_name=''  intf_description=''  default_value=0  timing_constraint=None  locs_specified=off  LOCs={}  io_standard={}  inherit_from_input=off  hdl_port=on  dbl_ovrd=off  block_type=gatewayin
  toDsp_config0 : xbsIndex_r4/Gateway In  gui_display_data_type=Fixed-point  arith_type=Unsigned  n_bits=32  bin_pt=0  preci_type=Single  exp_width=8  frac_width=24  rows=1  columns=1  quantization=Truncate  overflow=Wrap  period=Tclk*Naxi  UseAsADC=off  ADCChannel='1'  interface=AXI4-Lite  automatic_assignment=off  address_offset=hex2dec('800')  intf_name=''  intf_description=''  default_value=0  timing_constraint=None  locs_specified=off  LOCs={}  io_standard={}  inherit_from_input=off  hdl_port=on  dbl_ovrd=off  block_type=gatewayin
  toDsp_config1 : xbsIndex_r4/Gateway In  gui_display_data_type=Fixed-point  arith_type=Unsigned  n_bits=32  bin_pt=0  preci_type=Single  exp_width=8  frac_width=24  rows=1  columns=1  quantization=Truncate  overflow=Wrap  period=Tclk*Naxi  UseAsADC=off  ADCChannel='1'  interface=AXI4-Lite  automatic_assignment=off  address_offset=hex2dec('804')  intf_name=''  intf_description=''  default_value=0  timing_constraint=None  locs_specified=off  LOCs={}  io_standard={}  inherit_from_input=off  hdl_port=on  dbl_ovrd=off  block_type=gatewayin
  toDsp_config10 : xbsIndex_r4/Gateway In  gui_display_data_type=Fixed-point  arith_type=Unsigned  n_bits=32  bin_pt=0  preci_type=Single  exp_width=8  frac_width=24  rows=1  columns=1  quantization=Truncate  overflow=Wrap  period=Tclk*Naxi  UseAsADC=off  ADCChannel='1'  interface=AXI4-Lite  automatic_assignment=off  address_offset=hex2dec('828')  intf_name=''  intf_description=''  default_value=0  timing_constraint=None  locs_specified=off  LOCs={}  io_standard={}  inherit_from_input=off  hdl_port=on  dbl_ovrd=off  block_type=gatewayin
  toDsp_config11 : xbsIndex_r4/Gateway In  gui_display_data_type=Fixed-point  arith_type=Unsigned  n_bits=32  bin_pt=0  preci_type=Single  exp_width=8  frac_width=24  rows=1  columns=1  quantization=Truncate  overflow=Wrap  period=Tclk*Naxi  UseAsADC=off  ADCChannel='1'  interface=AXI4-Lite  automatic_assignment=off  address_offset=hex2dec('82c')  intf_name=''  intf_description=''  default_value=0  timing_constraint=None  locs_specified=off  LOCs={}  io_standard={}  inherit_from_input=off  hdl_port=on  dbl_ovrd=off  block_type=gatewayin
  toDsp_config12 : xbsIndex_r4/Gateway In  gui_display_data_type=Fixed-point  arith_type=Unsigned  n_bits=32  bin_pt=0  preci_type=Single  exp_width=8  frac_width=24  rows=1  columns=1  quantization=Truncate  overflow=Wrap  period=Tclk*Naxi  UseAsADC=off  ADCChannel='1'  interface=AXI4-Lite  automatic_assignment=off  address_offset=hex2dec('830')  intf_name=''  intf_description=''  default_value=0  timing_constraint=None  locs_specified=off  LOCs={}  io_standard={}  inherit_from_input=off  hdl_port=on  dbl_ovrd=off  block_type=gatewayin
  toDsp_config13 : xbsIndex_r4/Gateway In  gui_display_data_type=Fixed-point  arith_type=Unsigned  n_bits=32  bin_pt=0  preci_type=Single  exp_width=8  frac_width=24  rows=1  columns=1  quantization=Truncate  overflow=Wrap  period=Tclk*Naxi  UseAsADC=off  ADCChannel='1'  interface=AXI4-Lite  automatic_assignment=off  address_offset=hex2dec('834')  intf_name=''  intf_description=''  default_value=0  timing_constraint=None  locs_specified=off  LOCs={}  io_standard={}  inherit_from_input=off  hdl_port=on  dbl_ovrd=off  block_type=gatewayin
  toDsp_config2 : xbsIndex_r4/Gateway In  gui_display_data_type=Fixed-point  arith_type=Unsigned  n_bits=32  bin_pt=12  preci_type=Single  exp_width=8  frac_width=24  rows=1  columns=1  quantization=Truncate  overflow=Wrap  period=Tclk*Naxi  UseAsADC=off  ADCChannel='1'  interface=AXI4-Lite  automatic_assignment=off  address_offset=hex2dec('808')  intf_name=''  intf_description=''  default_value=0  timing_constraint=None  locs_specified=off  LOCs={}  io_standard={}  inherit_from_input=off  hdl_port=on  dbl_ovrd=off  block_type=gatewayin
  toDsp_config3 : xbsIndex_r4/Gateway In  gui_display_data_type=Fixed-point  arith_type=Unsigned  n_bits=32  bin_pt=0  preci_type=Single  exp_width=8  frac_width=24  rows=1  columns=1  quantization=Truncate  overflow=Wrap  period=Tclk*Naxi  UseAsADC=off  ADCChannel='1'  interface=AXI4-Lite  automatic_assignment=off  address_offset=hex2dec('80c')  intf_name=''  intf_description=''  default_value=0  timing_constraint=None  locs_specified=off  LOCs={}  io_standard={}  inherit_from_input=off  hdl_port=on  dbl_ovrd=off  block_type=gatewayin
  toDsp_config4 : xbsIndex_r4/Gateway In  gui_display_data_type=Fixed-point  arith_type=Unsigned  n_bits=32  bin_pt=0  preci_type=Single  exp_width=8  frac_width=24  rows=1  columns=1  quantization=Truncate  overflow=Wrap  period=Tclk*Naxi  UseAsADC=off  ADCChannel='1'  interface=AXI4-Lite  automatic_assignment=off  address_offset=hex2dec('810')  intf_name=''  intf_description=''  default_value=0  timing_constraint=None  locs_specified=off  LOCs={}  io_standard={}  inherit_from_input=off  hdl_port=on  dbl_ovrd=off  block_type=gatewayin
  toDsp_config5 : xbsIndex_r4/Gateway In  gui_display_data_type=Fixed-point  arith_type=Unsigned  n_bits=32  bin_pt=0  preci_type=Single  exp_width=8  frac_width=24  rows=1  columns=1  quantization=Truncate  overflow=Wrap  period=Tclk*Naxi  UseAsADC=off  ADCChannel='1'  interface=AXI4-Lite  automatic_assignment=off  address_offset=hex2dec('814')  intf_name=''  intf_description=''  default_value=0  timing_constraint=None  locs_specified=off  LOCs={}  io_standard={}  inherit_from_input=off  hdl_port=on  dbl_ovrd=off  block_type=gatewayin
  toDsp_config6 : xbsIndex_r4/Gateway In  gui_display_data_type=Fixed-point  arith_type=Unsigned  n_bits=32  bin_pt=0  preci_type=Single  exp_width=8  frac_width=24  rows=1  columns=1  quantization=Truncate  overflow=Wrap  period=Tclk*Naxi  UseAsADC=off  ADCChannel='1'  interface=AXI4-Lite  automatic_assignment=off  address_offset=hex2dec('818')  intf_name=''  intf_description=''  default_value=0  timing_constraint=None  locs_specified=off  LOCs={}  io_standard={}  inherit_from_input=off  hdl_port=on  dbl_ovrd=off  block_type=gatewayin
  toDsp_config7 : xbsIndex_r4/Gateway In  gui_display_data_type=Fixed-point  arith_type="Signed  (2's comp)"  n_bits=32  bin_pt=0  preci_type=Single  exp_width=8  frac_width=24  rows=1  columns=1  quantization=Truncate  overflow=Wrap  period=Tclk*Naxi  UseAsADC=off  ADCChannel='1'  interface=AXI4-Lite  automatic_assignment=off  address_offset=hex2dec('81c')  intf_name=''  intf_description=''  default_value=0  timing_constraint=None  locs_specified=off  LOCs={}  io_standard={}  inherit_from_input=off  hdl_port=on  dbl_ovrd=off  block_type=gatewayin
  toDsp_config8 : xbsIndex_r4/Gateway In  gui_display_data_type=Fixed-point  arith_type=Unsigned  n_bits=32  bin_pt=0  preci_type=Single  exp_width=8  frac_width=24  rows=1  columns=1  quantization=Truncate  overflow=Wrap  period=Tclk*Naxi  UseAsADC=off  ADCChannel='1'  interface=AXI4-Lite  automatic_assignment=off  address_offset=hex2dec('820')  intf_name=''  intf_description=''  default_value=0  timing_constraint=None  locs_specified=off  LOCs={}  io_standard={}  inherit_from_input=off  hdl_port=on  dbl_ovrd=off  block_type=gatewayin
  toDsp_config9 : xbsIndex_r4/Gateway In  gui_display_data_type=Fixed-point  arith_type=Unsigned  n_bits=32  bin_pt=0  preci_type=Single  exp_width=8  frac_width=24  rows=1  columns=1  quantization=Truncate  overflow=Wrap  period=Tclk*Naxi  UseAsADC=off  ADCChannel='1'  interface=AXI4-Lite  automatic_assignment=off  address_offset=hex2dec('824')  intf_name=''  intf_description=''  default_value=0  timing_constraint=None  locs_specified=off  LOCs={}  io_standard={}  inherit_from_input=off  hdl_port=on  dbl_ovrd=off  block_type=gatewayin
  tag scope: Ampl0=global, Ampl1=global, BW=global, ConfigReg0=global, FBen=global, FBgain=global, FBlimit=global, FBreset=global, FFgain=global, FFpolarity=global, Mfr=global, NotchSimEn=global, Nquad=global, Nsynch=global, RFen=global, RefSource=global, dFsb=global, debugMux=global, fbPolarity=global, fluxRampPhaseSetpoint=global, monitorChannel=global, omegaTsDf=global, omegaTsPhiRef=global, refDel=global, synchThresh=global, whiteNoiseGen=global
  wires:
  config0/1 -> toDsp_config0/1
  toDsp_config0/1 -> Register2/1
  config4/1 -> toDsp_config4/1
  toDsp_config4/1 -> Register3/1
  config5/1 -> toDsp_config5/1
  toDsp_config5/1 -> Register4/1
  config63/1 -> toDsp_cmd0/1
  toDsp_cmd0/1 -> Register6/1
  Register3/1 -> Slice6/1, Slice5/1
  Register6/1 -> Slice11/1, Slice4/1
  Slice5/1 -> Reinterpret/1
  Slice6/1 -> Reinterpret1/1
  Register4/1 -> BitBasher13/1, BitBasher12/1
  Slice1/1 -> [RefSource]
  Slice/1 -> [RFen]
  Slice2/1 -> [NotchSimEn]
  Slice3/1 -> [whiteNoiseGen]
  Reinterpret/1 -> [Ampl0]
  Reinterpret1/1 -> [Ampl1]
  Gateway Out6/1 -> Control Reg/1
  Slice4/1 -> [FBreset]
  BitBasher13/1 -> [dFsb]
  BitBasher12/1 -> [FBlimit]
  [NotchSimEn] -> Terminator2/1
  Slice9/1 -> [monitorChannel]
  config1/1 -> toDsp_config1/1
  toDsp_config1/1 -> Register12/1
  config2/1 -> toDsp_config2/1
  toDsp_config2/1 -> Register13/1
  config3/1 -> toDsp_config3/1
  toDsp_config3/1 -> Register14/1
  Slice12/1 -> [FBen]
  Register12/1 -> Slice12/1
  BitBasher15/1 -> [FBgain]
  Register13/1 -> BitBasher15/1
  Slice14/1 -> [refDel]
  Register14/1 -> Slice14/1
  config6/1 -> toDsp_config6/1
  toDsp_config6/1 -> Register15/1
  Register15/1 -> BitBasher16/1
  Slice7/1 -> [fbPolarity]
  [RefSource] -> Terminator1/1
  Slice8/1 -> [debugMux]
  BitBasher16/1 -> [BW]
  toDsp_config8/1 -> Register1/1
  Register1/1 -> BitBasher17/1, BitBasher18/1
  BitBasher17/1 -> [omegaTsPhiRef]
  BitBasher18/1 -> [omegaTsDf]
  config8/1 -> toDsp_config8/1
  toDsp_config7/1 -> Register7/1
  Register7/1 -> BitBasher19/1
  config7/1 -> toDsp_config7/1
  BitBasher19/1 -> [synchThresh]
  [ConfigReg0] -> Terminator/1
  toDsp_config9/1 -> Register8/1
  Register8/1 -> BitBasher20/1
  BitBasher20/1 -> Gateway Out1/1, [Mfr]
  config9/1 -> toDsp_config9/1
  toDsp_config10/1 -> Register9/1
  Register9/1 -> BitBasher21/1
  BitBasher21/1 -> [FFgain]
  config10/1 -> toDsp_config10/1
  toDsp_config11/1 -> Register10/1
  Register10/1 -> BitBasher22/1
  config11/1 -> toDsp_config11/1
  toDsp_config12/1 -> Register11/1
  Register11/1 -> BitBasher23/1
  BitBasher23/1 -> [Nsynch]
  config12/1 -> toDsp_config12/1
  [Nsynch] -> Terminator3/1
  BitBasher22/1 -> Shift/1
  Shift/1 -> [Nquad]
  [Nquad] -> Terminator4/1
  toDsp_config13/1 -> Register5/1
  Register5/1 -> BitBasher1/1
  BitBasher1/1 -> Gateway Out/1, [fluxRampPhaseSetpoint]
  config13/1 -> toDsp_config13/1
  Slice10/1 -> [FFpolarity]
  Gateway Out/1 -> Display/1
  Gateway Out1/1 -> Display1/1
  sigGenStart/1 -> Terminator5/1
  Slice11/1 -> sigGenStart/1
  Register2/1 -> Up Sample/1
  Up Sample/1 -> [ConfigReg0], Gateway Out6/1, Slice/1, Slice1/1, Slice2/1, Slice3/1, Slice7/1, Slice10/1, Slice8/1, Slice9/1

== system CryoDetXray/DspCore/DAC format ==
  note: Format DAC words (top)
      | create complex output stream for simulation (bottom)
  note: create an edge to synchronize DAC interleaver simulation to generate realtime DAC output for Simulink
  note: DAC outputs
  In1 : Inport
  BitBasher1 : xbsIndex_r4/BitBasher  bitexpr=|  display_expr=on  sr_1=Dac1  arith_type1=Unsigned  bin_pt1=0  sr_2=Dac0  arith_type2=Unsigned  bin_pt2=0  sr_3=Dac0  arith_type3=Unsigned  bin_pt3=0  sr_4=4  arith_type4=Unsigned  bin_pt4=0  dbl_ovrd=off  block_type=bitbasher
      | Dac1 = {I1,I0}
      | Dac0 = {Q1,Q0}
  Bus Selector : BusSelector  OutputSignals=I0,I1,Q0,Q1
  DAC demux clock : Subsystem
  Real-Imag to Complex : RealImagToComplex
  Register{,1..3} (4 alike) : xbsIndex_r4/Register  init=0  rst=off  en=off  dbl_ovrd=off  block_type=register
  Switch : Switch  Criteria=u2 > Threshold  Threshold=0.5
  Switch2 : Switch  Criteria=u2 > Threshold  Threshold=0.5
  i0 : xbsIndex_r4/Gateway Out  inherit_from_input=off  hdl_port=off  rows=1  columns=1  UseAsDAC=off  DACChannel='1'  interface=None  automatic_assignment=on  address_offset=hex2dec('00')  intf_name=''  intf_description=''  timing_constraint=None  locs_specified=off  LOCs={}  io_standard={}  block_type=gatewayout
  i1 : xbsIndex_r4/Gateway Out  inherit_from_input=off  hdl_port=off  rows=1  columns=1  UseAsDAC=off  DACChannel='1'  interface=None  automatic_assignment=on  address_offset=hex2dec('00')  intf_name=''  intf_description=''  timing_constraint=None  locs_specified=off  LOCs={}  io_standard={}  block_type=gatewayout
  q0 : xbsIndex_r4/Gateway Out  inherit_from_input=off  hdl_port=off  rows=1  columns=1  UseAsDAC=off  DACChannel='1'  interface=None  automatic_assignment=on  address_offset=hex2dec('00')  intf_name=''  intf_description=''  timing_constraint=None  locs_specified=off  LOCs={}  io_standard={}  block_type=gatewayout
  q1 : xbsIndex_r4/Gateway Out  inherit_from_input=off  hdl_port=off  rows=1  columns=1  UseAsDAC=off  DACChannel='1'  interface=None  automatic_assignment=on  address_offset=hex2dec('00')  intf_name=''  intf_description=''  timing_constraint=None  locs_specified=off  LOCs={}  io_standard={}  block_type=gatewayout
  dac0 : Outport
  dac1 : Outport  Port=2
  DACsim : Outport  Port=3
  wires:
  In1/1 -> Bus Selector/1
  BitBasher1/1 -> Register/1
  BitBasher1/2 -> Register2/1
  Real-Imag to Complex/1 -> DACsim/1
  q0/1 -> Switch/3
  i0/1 -> Switch/1
  i1/1 -> Switch2/1
  q1/1 -> Switch2/3
  DAC demux clock/1(IQtoggle) -> Switch2/2, Switch/2
  Switch/1 -> Real-Imag to Complex/1
  Switch2/1 -> Real-Imag to Complex/2
  Bus Selector/1 -> i0/1, BitBasher1/1  "<I0>"
  Bus Selector/2 -> q0/1, BitBasher1/2  "<I1>"
  Bus Selector/3 -> i1/1, BitBasher1/3  "<Q0>"
  Bus Selector/4 -> DAC demux clock/1(In1), q1/1, BitBasher1/4  "<Q1>"
  Register/1 -> Register1/1
  Register1/1 -> dac1/1
  Register2/1 -> Register3/1
  Register3/1 -> dac0/1
